simulink subsystem "Converter"  (R2023a)
settings: Solver=VariableStepAuto  StartTime=0.0  StopTime=10.0  RelTol=1e-3
undefined symbols (not defined in the file): Kku
settings Model: Creator=ycheb  LastModifiedBy=ycheb

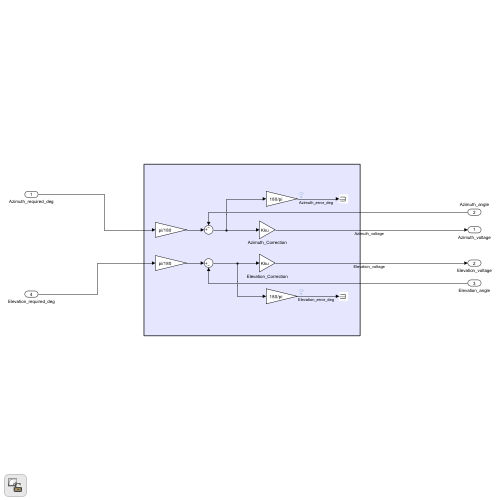
[thumbnail: Simulink's stored preview of the top-level diagram]
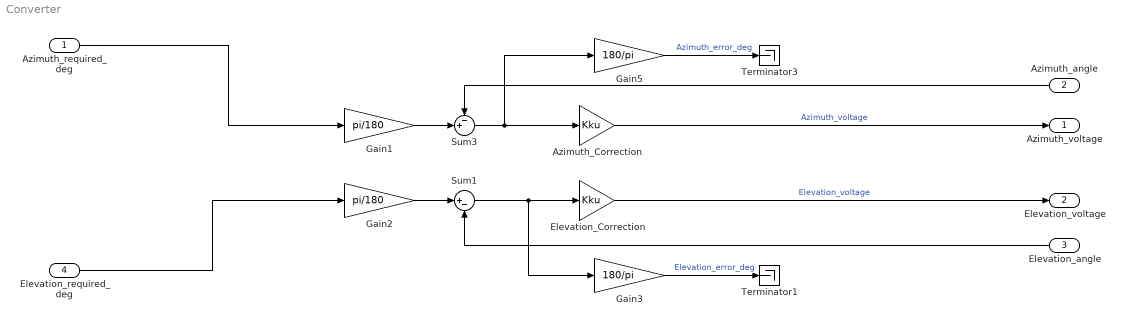
== system Converter ==
  Azimuth_required_deg : Inport
  Azimuth_angle : Inport  Port=2
  Elevation_angle : Inport  Port=3
  Elevation_required_deg : Inport  Port=4
  Azimuth_Correction : Gain  Gain=Kku
  Elevation_Correction : Gain  Gain=Kku
  Gain1 : Gain  Gain=pi/180
  Gain2 : Gain  Gain=pi/180
  Gain3 : Gain  Gain=180/pi
  Gain5 : Gain  Gain=180/pi
  Sum1 : Sum  Inputs=|+-
  Sum3 : Sum  Inputs=-+|
  Terminator1 : Terminator
  Terminator3 : Terminator
  Azimuth_voltage : Outport
  Elevation_voltage : Outport  Port=2
  wires:
  Gain2/1 -> Sum1/1
  Sum3/1 -> Azimuth_Correction/1, Gain5/1
  Gain5/1 -> Terminator3/1  "Azimuth_error_deg"
  Sum1/1 -> Elevation_Correction/1, Gain3/1
  Gain1/1 -> Sum3/2
  Azimuth_angle/1 -> Sum3/1
  Gain3/1 -> Terminator1/1  "Elevation_error_deg"
  Azimuth_required_deg/1 -> Gain1/1
  Elevation_angle/1 -> Sum1/2
  Azimuth_Correction/1 -> Azimuth_voltage/1  "Azimuth_voltage"
  Elevation_required_deg/1 -> Gain2/1
  Elevation_Correction/1 -> Elevation_voltage/1  "Elevation_voltage"
